simulink library "pi_ctrl"  (R2025b)
settings: Solver=VariableStepAuto  StartTime=0.0  StopTime=10.0  RelTol=1e-3
settings Model: Creator=dbagn  LastModifiedBy=dbagn

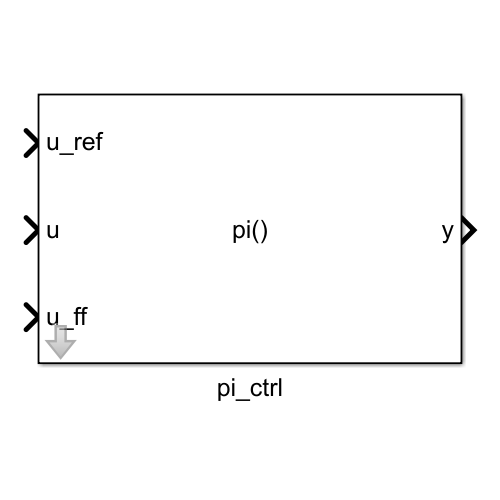
[thumbnail: Simulink's stored preview of the top-level diagram]
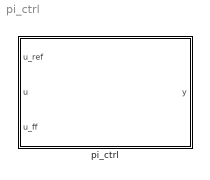
== system pi_ctrl ==
  pi_ctrl : Subsystem  mask{kp=0.5, ki=18, ts=125e-6, lim_up=1, lim_down=-1}
      mask Display:
      | disp('pi()');
      | port_label('input', 1, 'u_ref');
      | port_label('input', 2, 'u');
      | port_label('input', 3, 'u_ff');
      | port_label('output', 1, 'y');

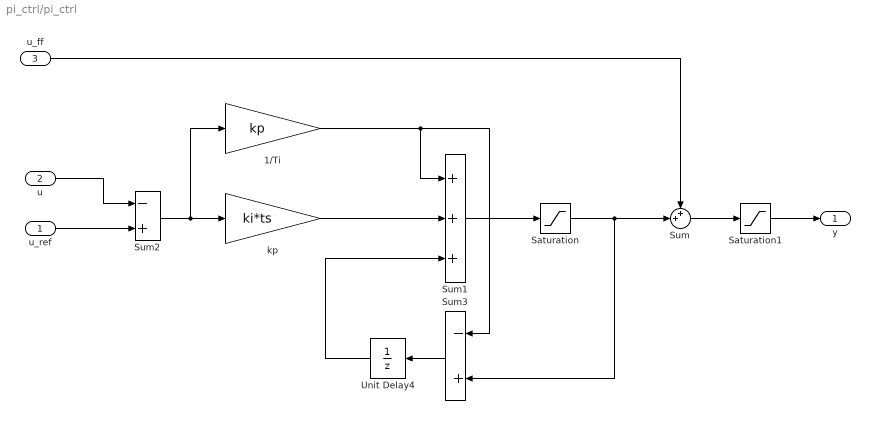
== system pi_ctrl/pi_ctrl ==
  u_ref : Inport
  u : Inport  Port=2
  u_ff : Inport  Port=3
  1/Ti : Gain  Gain=kp  SaturateOnIntegerOverflow=on  OutDataTypeStr=Inherit: Same as input  ParamDataTypeStr=Inherit: Same as input
  Saturation : Saturate  UpperLimit=lim_up  LowerLimit=lim_down
  Saturation1 : Saturate  UpperLimit=lim_up  LowerLimit=lim_down
  Sum : Sum  Inputs=++|
  Sum1 : Sum  Inputs=+++  SaturateOnIntegerOverflow=on
  Sum2 : Sum  Inputs=-+  SaturateOnIntegerOverflow=on
  Sum3 : Sum  Inputs=-+  SaturateOnIntegerOverflow=on
  Unit Delay4 : UnitDelay  SampleTime=-1  HasFrameUpgradeWarning=on
  kp : Gain  Gain=ki*ts  SaturateOnIntegerOverflow=on  OutDataTypeStr=Inherit: Same as input  ParamDataTypeStr=Inherit: Same as input
  y : Outport
  wires:
  1/Ti/1 -> Sum1/1, Sum3/1
  Sum3/1 -> Unit Delay4/1
  Unit Delay4/1 -> Sum1/3
  u_ref/1 -> Sum2/2
  u/1 -> Sum2/1
  Sum2/1 -> kp/1, 1/Ti/1
  Saturation/1 -> Sum/2, Sum3/2
  kp/1 -> Sum1/2
  Sum1/1 -> Saturation/1
  u_ff/1 -> Sum/1
  Saturation1/1 -> y/1
  Sum/1 -> Saturation1/1
